simulink model "untitled2"  (R2012b)
settings: Solver=ode45  StartTime=0.0  StopTime=10.0  RelTol=1e-3
settings Model: Creator=Vicon CS  LastModifiedBy=Vicon CS

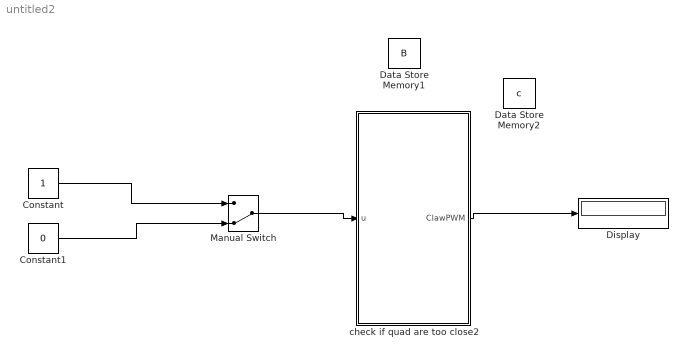
== system untitled2 ==
  Constant : Constant
  Constant1 : Constant  Value=0
  Data Store Memory1 : DataStoreMemory  DataStoreName=B  OutDataTypeStr=int8
  Data Store Memory2 : DataStoreMemory  DataStoreName=c  OutDataTypeStr=int8
  Display : Display
  Manual Switch : ManualSwitch  CurrentSetting=0
  check if quad are too close2 : MATLAB Function  TreatAsAtomicUnit=on
  wires:
  check if quad are too close2/1(ClawPWM) -> Display/1
  Manual Switch/1 -> check if quad are too close2/1(u)
  Constant/1 -> Manual Switch/1
  Constant1/1 -> Manual Switch/2

== matlab function untitled2/check if quad are too close2 ==
  data: u input; ClawPWM output; B data_store_memory; c data_store_memory; B1 data_store_memory; B2 data_store_memory
function ClawPWM = CLAW(u)
global B;
global c;

if(u==1)
    B = B + 1;
    if(mod(B,2)>0)
        c = 1200;
        ClawPWM = 1200;
    else
        c = 1690;
        ClawPWM = 1690;
    end

else
    ClawPWM = c;
end
   
end
